simulink model "T1"  (R2022b)
settings: Solver=ode45  StartTime=0.0  StopTime=10.0  MaxStep=0.0001  RelTol=1e-3
values from neighbouring files (symbols this model uses):
  g = 9.81    [Parametros_T1.m]
  l1 = 0.3    [Parametros_T1.m]
  l2 = 0.25    [Parametros_T1.m]
  m1 = 0.2    [Parametros_T1.m]
  m2 = 0.1    [Parametros_T1.m]
settings Model: Creator=edgar  LastModifiedBy=mluser
settings ModelReferenceCC: EnableRefExpFcnMdlSchedulingChecks=on

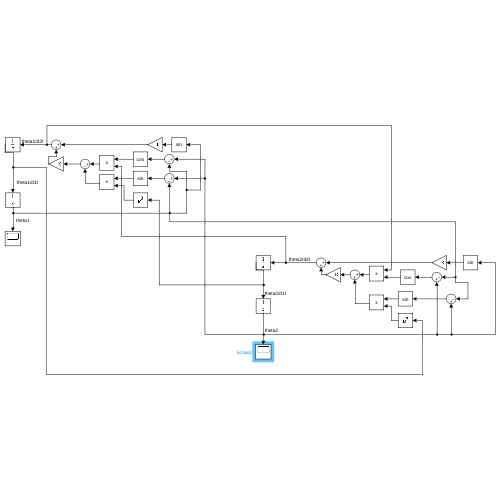
[thumbnail: Simulink's stored preview of the top-level diagram]
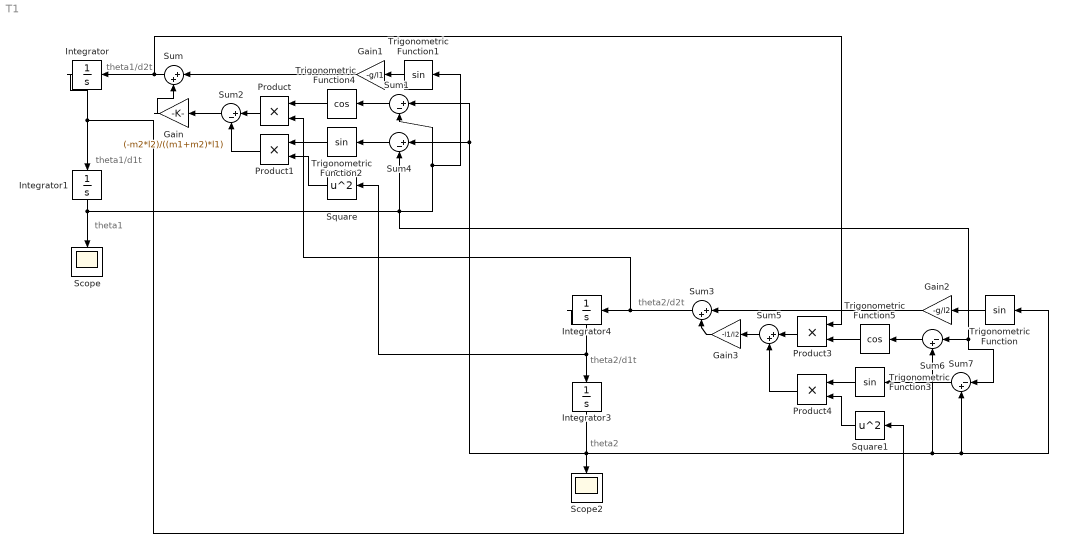
== system T1 ==
  note: theta1
  note: theta1/d2t
  note: theta1/d1t
  note: theta2/d2t
  note: theta2/d1t
  note: theta2
  Gain : Gain  Gain=(-m2*l2)/((m1+m2)*l1)
  Gain1 : Gain  Gain=-g/l1
  Gain2 : Gain  Gain=-g/l2
  Gain3 : Gain  Gain=-l1/l2
  Integrator : Integrator
  Integrator1 : Integrator
  Integrator3 : Integrator  InitialCondition=(35*pi)/180
  Integrator4 : Integrator
  Product{,1,3..4} (4 alike) : Product
  Scope : Scope
  Scope2 : Scope
  Square : Math  Operator=square
  Square1 : Math  Operator=square
  Sum : Sum  Inputs=|++
  Sum1 : Sum  Inputs=|+-
  Sum2 : Sum  Inputs=|+-
  Sum3 : Sum  Inputs=|++
  Sum4 : Sum  Inputs=|+-
  Sum5 : Sum  Inputs=|++
  Sum6 : Sum  Inputs=|-+
  Sum7 : Sum  Inputs=|-+
  Trigonometric Function{,1..3} (4 alike) : Trigonometry
  Trigonometric Function4 : Trigonometry  Operator=cos
  Trigonometric Function5 : Trigonometry  Operator=cos
  wires:
  Integrator1/1 -> Scope/1, Sum7/1, Sum6/1, Trigonometric Function1/1, Sum1/2, Sum4/2
  Integrator/1 -> Square1/1, Integrator1/1
  Sum/1 -> Product3/1, Integrator/1
  Gain1/1 -> Sum/1
  Trigonometric Function1/1 -> Gain1/1
  Trigonometric Function4/1 -> Product/1
  Integrator3/1 -> Sum6/2, Trigonometric Function/1, Sum7/2, Sum4/1, Sum1/1, Scope2/1
  Integrator4/1 -> Square/1, Integrator3/1
  Sum1/1 -> Trigonometric Function4/1
  Square/1 -> Product1/2
  Sum3/1 -> Product/2, Integrator4/1
  Trigonometric Function2/1 -> Product1/1
  Sum4/1 -> Trigonometric Function2/1
  Gain2/1 -> Sum3/1
  Trigonometric Function/1 -> Gain2/1
  Gain3/1 -> Sum3/2
  Sum5/1 -> Gain3/1
  Product3/1 -> Sum5/1
  Product4/1 -> Sum5/2
  Trigonometric Function5/1 -> Product3/2
  Sum6/1 -> Trigonometric Function5/1
  Trigonometric Function3/1 -> Product4/1
  Sum7/1 -> Trigonometric Function3/1
  Gain/1 -> Sum/2
  Sum2/1 -> Gain/1
  Product1/1 -> Sum2/2
  Product/1 -> Sum2/1
  Square1/1 -> Product4/2
